simulink model "propeller_start"  (R2021b)
settings: Solver=VariableStepAuto  StartTime=0.0  StopTime=10.0  RelTol=1e-3
settings Model: Creator=cirie  LastModifiedBy=cirie

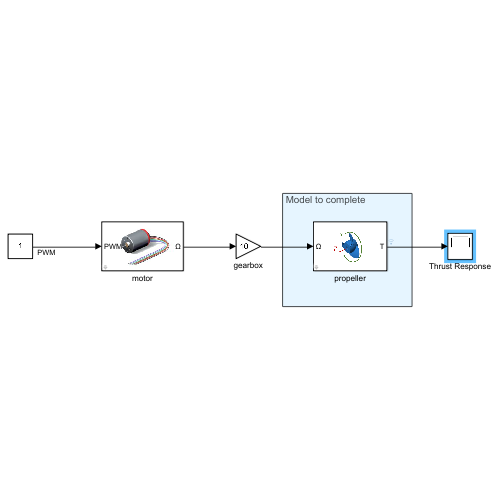
[thumbnail: Simulink's stored preview of the top-level diagram]
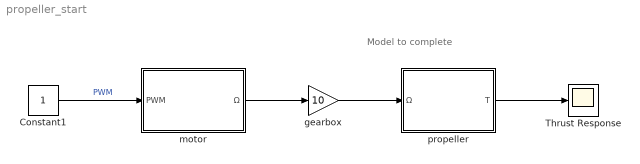
== system propeller_start ==
  note: Model to complete
  Constant1 : Constant
  Thrust Response : Scope
  gearbox : Gain  Gain=10
  motor : Subsystem  mask(DC Motor){J=1e-4, km=0.1, R=1, Vmax=7.2}
      mask prompts: J "Inertia, J [kgm^2]"; km "Motor constant, km [V*s/rad]"; R "Resistance, R [Ohm]"; Vmax "Maximum Voltage, Vmax [V]"
      mask help:
      | Circuit Dynamics:   PWM*Vmax == I*R + km*Ω
      | Rotor Dynamics:     J*dΩ/dt == km*I
      mask Display: image('$imagefile'); % Use "Edit Image" on toolstrip to change.
  propeller : Subsystem  mask(Propeller Model){D=0.1, kt=0.01, rho=1000}
      mask prompts: D "Propeller Diameter [m]"; kt "Thrust Coefficient"; rho "Fluid density [kg/m^3]"
      mask help: Propeller Dynamics: T = kt*rho*omega^2*D^4
      mask Display: image('$imagefile'); % Use "Edit Image" on toolstrip to change.
  wires:
  propeller/1(T) -> Thrust Response/1
  Constant1/1 -> motor/1(PWM)  "PWM"
  motor/1(Ω) -> gearbox/1
  gearbox/1 -> propeller/1(Ω)

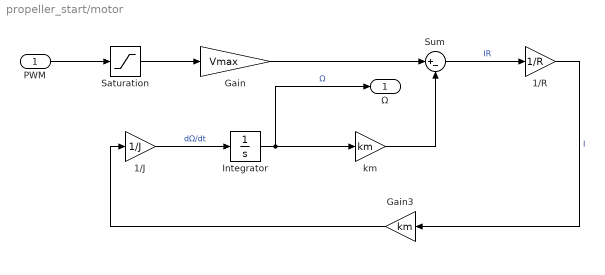
== system propeller_start/motor ==
  PWM : Inport
  1/J : Gain  Gain=1/J
  1/R : Gain  Gain=1/R
  Gain : Gain  Gain=Vmax
  Gain3 : Gain  Gain=km
  Integrator : Integrator
  Saturation : Saturate  UpperLimit=1  LowerLimit=-1
  Sum : Sum  Inputs=|+-
  km : Gain  Gain=km
  Ω : Outport
  wires:
  1/J/1 -> Integrator/1  "dΩ/dt"
  Sum/1 -> 1/R/1  "IR"
  Integrator/1 -> Ω/1, km/1  "Ω"
  1/R/1 -> Gain3/1  "I"
  PWM/1 -> Saturation/1
  Gain/1 -> Sum/1
  Saturation/1 -> Gain/1
  Gain3/1 -> 1/J/1
  km/1 -> Sum/2

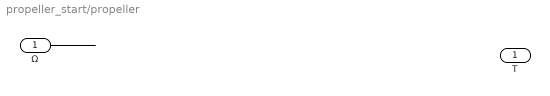
== system propeller_start/propeller ==
  Ω : Inport
  T : Outport
  wires:
  ? -> T/1  "T"
  Ω/1 -> ?
